simulink model "Desorbtion_mt"  (Simulink 9.2)
settings: Solver=ode3  StartTime=0.0  StopTime=20000  FixedStep=0.1  RelTol=1e-3  EnableMultiTasking=on
settings Model: Creator=User  LastModifiedBy=user
settings OptimizationCC: ExpressionDepthLimit=2147483647  InitFltsAndDblsToZero=on
settings DebuggingCC: SolverPrmCheckMsg=warning
settings ConfigComp: CovSFcnEnable=off

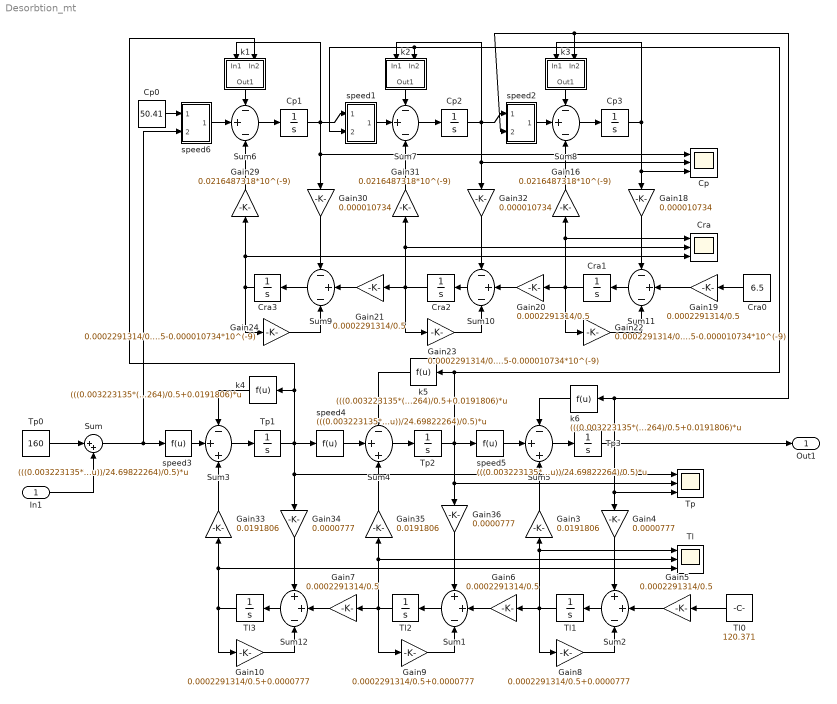
== system Desorbtion_mt ==
  In1 : Inport
  Cp : Scope  NumInputPorts=3
  Cp0 : Constant  Value=50.41
  Cp1 : Integrator  InitialCondition=62.8910352690798
  Cp2 : Integrator  InitialCondition=78.0581380338609
  Cp3 : Integrator  InitialCondition=97.0647284967471
  Cra : Scope  NumInputPorts=3
  Cra0 : Constant  Value=6.5
  Cra1 : Integrator  InitialCondition=4.2264294731348
  Cra2 : Integrator  InitialCondition=2.3980548949894
  Cra3 : Integrator  InitialCondition=0.9249430199510
  Gain10 : Gain  Gain=0.0002291314/0.5+0.0000777
  Gain16 : Gain  Gain=0.0216487318*10^(-9)
  Gain18 : Gain  Gain=0.000010734
  Gain{5..7,19..21} (6 alike) : Gain  Gain=0.0002291314/0.5
  Gain22 : Gain  Gain=0.0002291314/0.5-0.000010734*10^(-9)
  Gain23 : Gain  Gain=0.0002291314/0.5-0.000010734*10^(-9)
  Gain24 : Gain  Gain=0.0002291314/0.5-0.000010734*10^(-9)
  Gain29 : Gain  Gain=0.0216487318*10^(-9)
  Gain3 : Gain  Gain=0.0191806
  Gain30 : Gain  Gain=0.000010734
  Gain31 : Gain  Gain=0.0216487318*10^(-9)
  Gain32 : Gain  Gain=0.000010734
  Gain33 : Gain  Gain=0.0191806
  Gain34 : Gain  Gain=0.0000777
  Gain35 : Gain  Gain=0.0191806
  Gain36 : Gain  Gain=0.0000777
  Gain4 : Gain  Gain=0.0000777
  Gain8 : Gain  Gain=0.0002291314/0.5+0.0000777
  Gain9 : Gain  Gain=0.0002291314/0.5+0.0000777
  Sum : Sum  Inputs=|++
  Sum1 : Sum  Inputs=++-
  Sum{6..11} (6 alike) : Sum  Inputs=-+-
  Sum12 : Sum  Inputs=++-
  Sum2 : Sum  Inputs=++-
  Sum3 : Sum  Inputs=-++
  Sum4 : Sum  Inputs=-++
  Sum5 : Sum  Inputs=-++
  Tl : Scope  NumInputPorts=3
  Tl0 : Constant  Value=120.371
  Tl1 : Integrator  InitialCondition=124.7521008288133
  Tl2 : Integrator  InitialCondition=128.9747697447938
  Tl3 : Integrator  InitialCondition=133.0396819538713
  Tp : Scope  NumInputPorts=3
  Tp0 : Constant  Value=160
  Tp1 : Integrator  InitialCondition=157.0139168404367
  Tp2 : Integrator  InitialCondition=153.8794297307592
  Tp3 : Integrator  InitialCondition=150.5911681762652  IgnoreLimit=on
  k1 : Subsystem
  k2 : Subsystem
  k3 : Subsystem
  k4 : Fcn  Expr=(((0.003223135*(273+u))/24.69822264)/0.5+0.0191806)*u
  k5 : Fcn  Expr=(((0.003223135*(273+u))/24.69822264)/0.5+0.0191806)*u
  k6 : Fcn  Expr=(((0.003223135*(273+u))/24.69822264)/0.5+0.0191806)*u
  speed1 : Subsystem
  speed2 : Subsystem
  speed3 : Fcn  Expr=(((0.003223135*(273+u))/24.69822264)/0.5)*u
  speed4 : Fcn  Expr=(((0.003223135*(273+u))/24.69822264)/0.5)*u
  speed5 : Fcn  Expr=(((0.003223135*(273+u))/24.69822264)/0.5)*u
  speed6 : Subsystem
  Out1 : Outport
  wires:
  Sum6/1 -> Cp1/1
  speed1/1(Out1) -> Sum7/2
  Sum7/1 -> Cp2/1
  speed2/1(Out1) -> Sum8/2
  Sum8/1 -> Cp3/1
  Cp1/1 -> Gain30/1, Cp/1, speed1/1(In1), k1/1(In1)
  Cp2/1 -> Gain32/1, Cp/2, speed2/1(In1), k2/1(In1)
  Gain29/1 -> Sum6/3
  Cp3/1 -> Gain18/1, Cp/3, k3/1(In1)
  Gain31/1 -> Sum7/3
  Gain16/1 -> Sum8/3
  Gain30/1 -> Sum9/1
  Gain32/1 -> Sum10/1
  Gain18/1 -> Sum11/1
  Gain19/1 -> Sum11/2
  Sum11/1 -> Cra1/1
  Cra1/1 -> Gain22/1, Gain20/1, Gain16/1, Cra/1
  Gain20/1 -> Sum10/2
  Sum10/1 -> Cra2/1
  Cra2/1 -> Gain23/1, Gain21/1, Gain31/1, Cra/2
  Gain21/1 -> Sum9/2
  Sum9/1 -> Cra3/1
  Cra3/1 -> Gain24/1, Gain29/1, Cra/3
  Gain22/1 -> Sum11/3
  Gain23/1 -> Sum10/3
  Gain24/1 -> Sum9/3
  speed3/1 -> Sum3/2
  k4/1 -> Sum3/1
  Sum3/1 -> Tp1/1
  speed4/1 -> Sum4/2
  k5/1 -> Sum4/1
  Sum4/1 -> Tp2/1
  speed5/1 -> Sum5/2
  k6/1 -> Sum5/1
  Sum5/1 -> Tp3/1
  Tp1/1 -> Gain34/1, Tp/1, k4/1, k1/2(In2), speed4/1
  Tp2/1 -> Gain36/1, Tp/2, k5/1, speed1/2(In2), k2/2(In2), speed5/1
  Gain33/1 -> Sum3/3
  Tp3/1 -> Out1/1, k6/1, k3/2(In2), speed2/2(In2), Gain4/1, Tp/3
  Gain35/1 -> Sum4/3
  Gain3/1 -> Sum5/3
  Gain34/1 -> Sum12/1
  Gain36/1 -> Sum1/1
  Gain4/1 -> Sum2/1
  Gain5/1 -> Sum2/2
  Sum2/1 -> Tl1/1
  Tl1/1 -> Gain8/1, Gain6/1, Gain3/1, Tl/1
  Gain6/1 -> Sum1/2
  Sum1/1 -> Tl2/1
  Tl2/1 -> Gain9/1, Gain7/1, Gain35/1, Tl/2
  Gain7/1 -> Sum12/2
  Sum12/1 -> Tl3/1
  Tl3/1 -> Gain10/1, Gain33/1, Tl/3
  Gain8/1 -> Sum2/3
  Gain9/1 -> Sum1/3
  Gain10/1 -> Sum12/3
  Tp0/1 -> Sum/1
  speed6/1(Out1) -> Sum6/2
  Cp0/1 -> speed6/1(In1)
  k1/1(Out1) -> Sum6/1
  k2/1(Out1) -> Sum7/1
  k3/1(Out1) -> Sum8/1
  Cra0/1 -> Gain19/1
  Tl0/1 -> Gain5/1
  Sum/1 -> speed6/2(In2), speed3/1
  In1/1 -> Sum/2

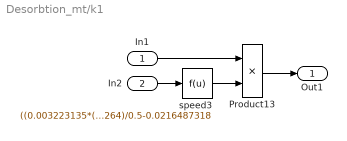
== system Desorbtion_mt/k1 ==
  In1 : Inport
  In2 : Inport  Port=2
  Product13 : Product  SaturateOnIntegerOverflow=on  InputSameDT=on  OutDataTypeStr=Inherit: Same as first input
  speed3 : Fcn  Expr=((0.003223135*(273+u))/24.69822264)/0.5-0.0216487318
  Out1 : Outport
  wires:
  Product13/1 -> Out1/1
  speed3/1 -> Product13/2
  In2/1 -> speed3/1
  In1/1 -> Product13/1

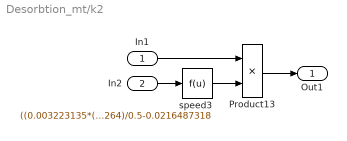
== system Desorbtion_mt/k2 ==
  In1 : Inport
  In2 : Inport  Port=2
  Product13 : Product  SaturateOnIntegerOverflow=on  InputSameDT=on  OutDataTypeStr=Inherit: Same as first input
  speed3 : Fcn  Expr=((0.003223135*(273+u))/24.69822264)/0.5-0.0216487318
  Out1 : Outport
  wires:
  In1/1 -> Product13/1
  In2/1 -> speed3/1
  speed3/1 -> Product13/2
  Product13/1 -> Out1/1

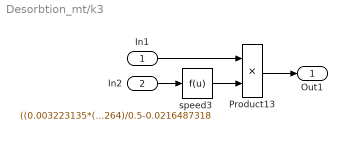
== system Desorbtion_mt/k3 ==
  In1 : Inport
  In2 : Inport  Port=2
  Product13 : Product  SaturateOnIntegerOverflow=on  InputSameDT=on  OutDataTypeStr=Inherit: Same as first input
  speed3 : Fcn  Expr=((0.003223135*(273+u))/24.69822264)/0.5-0.0216487318
  Out1 : Outport
  wires:
  Product13/1 -> Out1/1
  speed3/1 -> Product13/2
  In2/1 -> speed3/1
  In1/1 -> Product13/1

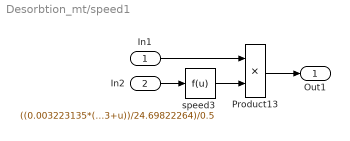
== system Desorbtion_mt/speed1 ==
  In1 : Inport
  In2 : Inport  Port=2
  Product13 : Product  SaturateOnIntegerOverflow=on  InputSameDT=on  OutDataTypeStr=Inherit: Same as first input
  speed3 : Fcn  Expr=((0.003223135*(273+u))/24.69822264)/0.5
  Out1 : Outport
  wires:
  Product13/1 -> Out1/1
  speed3/1 -> Product13/2
  In2/1 -> speed3/1
  In1/1 -> Product13/1

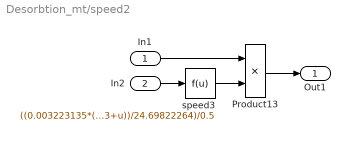
== system Desorbtion_mt/speed2 ==
  In1 : Inport
  In2 : Inport  Port=2
  Product13 : Product  SaturateOnIntegerOverflow=on  InputSameDT=on  OutDataTypeStr=Inherit: Same as first input
  speed3 : Fcn  Expr=((0.003223135*(273+u))/24.69822264)/0.5
  Out1 : Outport
  wires:
  In1/1 -> Product13/1
  In2/1 -> speed3/1
  speed3/1 -> Product13/2
  Product13/1 -> Out1/1

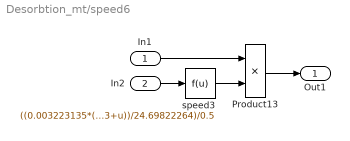
== system Desorbtion_mt/speed6 ==
  In1 : Inport
  In2 : Inport  Port=2
  Product13 : Product  SaturateOnIntegerOverflow=on  InputSameDT=on  OutDataTypeStr=Inherit: Same as first input
  speed3 : Fcn  Expr=((0.003223135*(273+u))/24.69822264)/0.5
  Out1 : Outport
  wires:
  In1/1 -> Product13/1
  In2/1 -> speed3/1
  speed3/1 -> Product13/2
  Product13/1 -> Out1/1
